simulink model "projekat2"  (R2021a)
settings: Solver=ode4  StartTime=0.0  StopTime=2000.0  FixedStep=0.1  RelTol=1e-3
undefined symbols (not defined in the file): Kd_cap, Kp, Kp_cap, Ku_cap, poremecaj, sel, sel1, Ti
libraries: cstblocks x2, fuzblock x1, eeGeneralControl x1
settings Model: Creator=svorc  LastModifiedBy=svorc

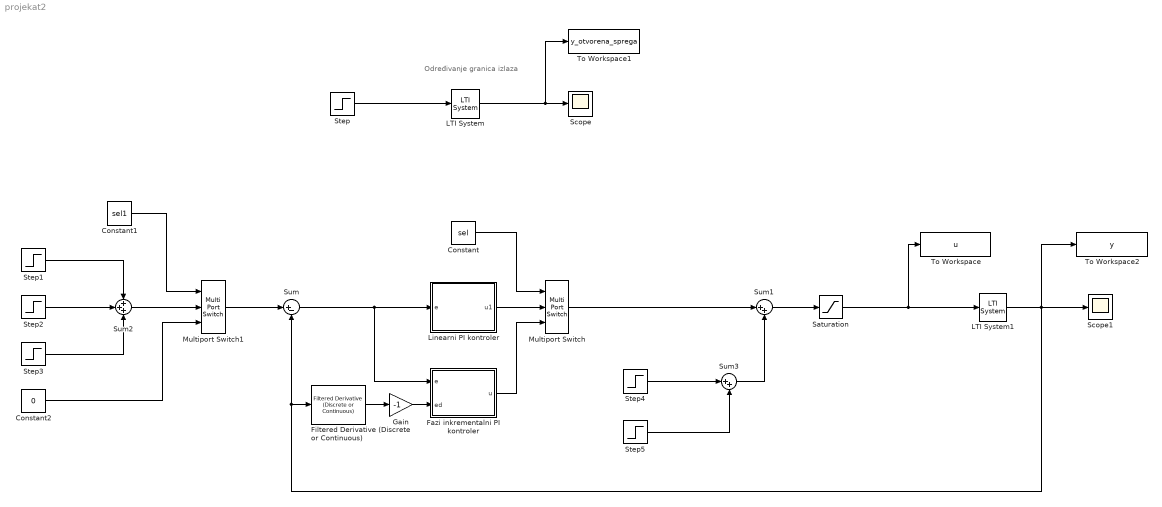
== system projekat2 ==
  note: Određivanje granica izlaza
  Constant : Constant  Value=sel
  Constant1 : Constant  Value=sel1
  Constant2 : Constant  Value=0
  Fazi inkrementalni PI kontroler : Subsystem
  Filtered Derivative (Discrete or Continuous) : eeGeneralControl/Filtered Derivative (Discrete or Continuous)  K=1  T=1  B=inf  A=-inf  minRatio=10  init_option=Inherited from block input  x0=0  Ts=-1
      settings: SourceProductBaseCode=PS
  Gain : Gain  Gain=-1
  LTI System : cstblocks/LTI System  sys=G  IC=[]
  LTI System1 : cstblocks/LTI System  sys=G  IC=[]
  Linearni PI kontroler : Subsystem
  Multiport Switch : MultiPortSwitch  Inputs=2
  Multiport Switch1 : MultiPortSwitch  Inputs=2
  Saturation : Saturate  UpperLimit=1.2  LowerLimit=-1.2
  Scope : Scope
  Scope1 : Scope
  Step : Step  Time=0  After=1.2  SampleTime=0
  Step1 : Step  Time=100  After=-2  SampleTime=0
  Step2 : Step  Time=500  After=4  SampleTime=0
  Step3 : Step  Time=1200  After=-2  SampleTime=0
  Step4 : Step  Time=100  After=poremecaj  SampleTime=0
  Step5 : Step  Time=1000  After=-2*poremecaj  SampleTime=0
  Sum : Sum  Inputs=|+-
  Sum1 : Sum  Inputs=|++
  Sum2 : Sum  Inputs=+++
  Sum3 : Sum  Inputs=|++
  To Workspace : ToWorkspace  VariableName=u  SampleTime=-1
  To Workspace1 : ToWorkspace  VariableName=y_otvorena_sprega  SampleTime=-1
  To Workspace2 : ToWorkspace  VariableName=y  SampleTime=-1
  wires:
  Step/1 -> LTI System/1
  LTI System/1 -> To Workspace1/1, Scope/1
  LTI System1/1 -> Sum/2, Filtered Derivative (Discrete or Continuous)/1, To Workspace2/1, Scope1/1
  Saturation/1 -> To Workspace/1, LTI System1/1
  Step1/1 -> Sum2/1
  Step2/1 -> Sum2/2
  Step3/1 -> Sum2/3
  Sum/1 -> Fazi inkrementalni PI kontroler/1(e), Linearni PI kontroler/1(e)
  Constant/1 -> Multiport Switch/1
  Linearni PI kontroler/1(u1) -> Multiport Switch/2
  Fazi inkrementalni PI kontroler/1(u) -> Multiport Switch/3
  Filtered Derivative (Discrete or Continuous)/1 -> Gain/1
  Gain/1 -> Fazi inkrementalni PI kontroler/2(ed)
  Sum2/1 -> Multiport Switch1/2
  Multiport Switch1/1 -> Sum/1
  Constant1/1 -> Multiport Switch1/1
  Constant2/1 -> Multiport Switch1/3
  Multiport Switch/1 -> Sum1/1
  Sum1/1 -> Saturation/1
  Sum3/1 -> Sum1/2
  Step4/1 -> Sum3/1
  Step5/1 -> Sum3/2

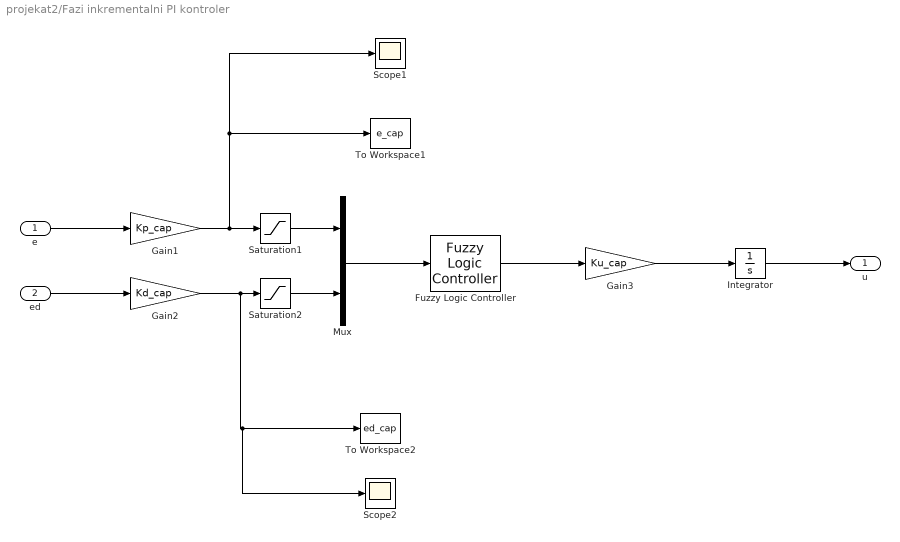
== system projekat2/Fazi inkrementalni PI kontroler ==
  e : Inport
  ed : Inport  Port=2
  Fuzzy Logic Controller : fuzblock/Fuzzy Logic  Controller  FIS='lin_fpd_blaga.fis'  OutputSampleNumber=101  DataType=double  FuzzifiedInputs=off  RuleFiringStrengths=off  RuleOutputs=off  AggregatedOutputs=off  SimulateUsing=Interpreted execution  OutOfRangeInputValueMessage=warning  NoRuleFiredMessage=warning  EmptyOutputFuzzySetMessage=warning
  Gain1 : Gain  Gain=Kp_cap  SaturateOnIntegerOverflow=on  OutDataTypeStr=Inherit: Same as input  ParamDataTypeStr=Inherit: Same as input
  Gain2 : Gain  Gain=Kd_cap  SaturateOnIntegerOverflow=on  OutDataTypeStr=Inherit: Same as input  ParamDataTypeStr=Inherit: Same as input
  Gain3 : Gain  Gain=Ku_cap  SaturateOnIntegerOverflow=on  OutDataTypeStr=Inherit: Same as input  ParamDataTypeStr=Inherit: Same as input
  Integrator : Integrator
  Mux : Mux  Inputs=2
  Saturation1 : Saturate  UpperLimit=1  LowerLimit=-1
  Saturation2 : Saturate  UpperLimit=1  LowerLimit=-1
  Scope1 : Scope
  Scope2 : Scope
  To Workspace1 : ToWorkspace  VariableName=e_cap  SampleTime=-1
  To Workspace2 : ToWorkspace  VariableName=ed_cap  SampleTime=-1
  u : Outport
  wires:
  Mux/1 -> Fuzzy Logic Controller/1
  Saturation2/1 -> Mux/2
  Saturation1/1 -> Mux/1
  e/1 -> Gain1/1
  ed/1 -> Gain2/1
  Gain3/1 -> Integrator/1
  Integrator/1 -> u/1
  Gain1/1 -> Scope1/1, To Workspace1/1, Saturation1/1
  Fuzzy Logic Controller/1 -> Gain3/1
  Gain2/1 -> To Workspace2/1, Scope2/1, Saturation2/1

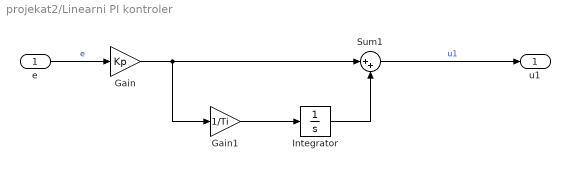
== system projekat2/Linearni PI kontroler ==
  e : Inport
  Gain : Gain  Gain=Kp
  Gain1 : Gain  Gain=1/Ti
  Integrator : Integrator
  Sum1 : Sum  Inputs=|++
  u1 : Outport
  wires:
  Gain/1 -> Sum1/1, Gain1/1
  e/1 -> Gain/1  "e"
  Integrator/1 -> Sum1/2
  Gain1/1 -> Integrator/1
  Sum1/1 -> u1/1  "u1"
